simulink model "DC_motor_with_nested_PID"  (R2013b)
settings: Solver=ode45  StartTime=0.0  StopTime=20  MaxStep=0.1  RelTol=1e-3
values from neighbouring files (symbols this model uses):
  J = 1.66e-5    (= 1.66e-05)    [RunMotorSim.m]    (also in RunMotorSim_OpenLoop.m)
  KD = 1.33e-8    (= 1.33e-08)    [RunMotorSim.m]    (also in RunMotorSim_OpenLoop.m)
  KT = 7.5e-3    (= 0.0075)    [RunMotorSim.m]    (also in RunMotorSim_OpenLoop.m)
  pow = 1.88    [RunMotorSim.m]    (also in RunMotorSim_OpenLoop.m = 2)
libraries: simulink x1
settings Model: Creator=aberger  LastModifiedBy=aberger
settings DataIOCC: MaxDataPoints=100000

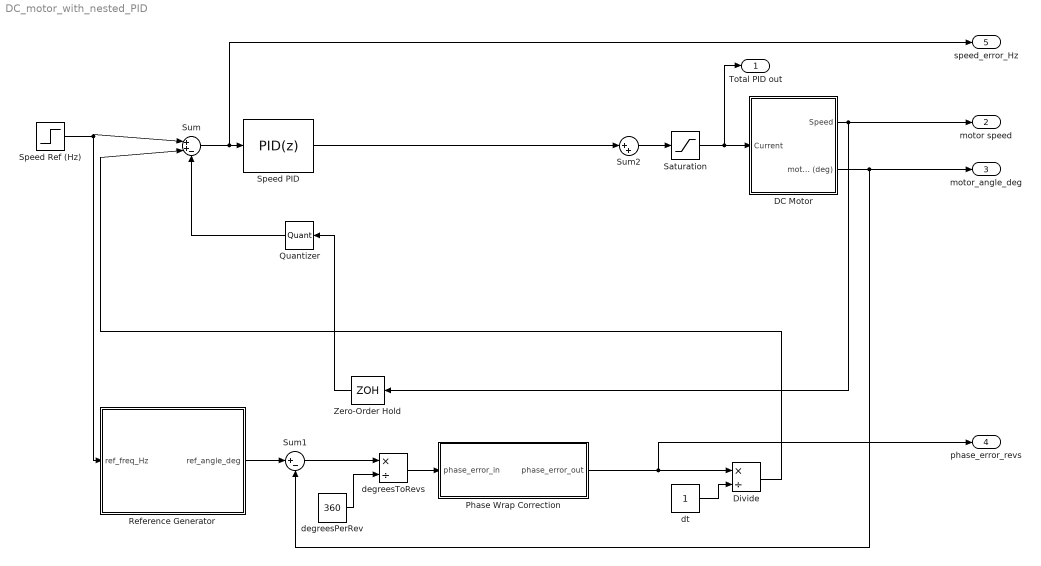
== system DC_motor_with_nested_PID ==
  DC Motor : Subsystem
  Divide : Product  Inputs=*/
  Phase Wrap Correction : Subsystem
  Quantizer : Quantizer  QuantizationInterval=.025
  Reference Generator : Subsystem
  Saturation : Saturate  UpperLimit=1  LowerLimit=0
  Speed PID : simulink/Continuous/PID Controller  Controller=PID  TimeDomain=Discrete-time  SampleTime=.001  IntegratorMethod=Forward Euler  FilterMethod=Forward Euler  Form=Parallel  P=0.4  I=.04  D=0  N=100  InitialConditionSource=internal  InitialConditionForIntegrator=0  InitialConditionForFilter=0  ExternalReset=none  LimitOutput=on  UpperSaturationLimit=1  LowerSaturationLimit=0  LinearizeAsGain=on  AntiWindupMode=none  Kb=1  TrackingMode=off  Kt=1  PParamMin=[]  PParamMax=[]  IParamMin=[]  IParamMax=[]  DParamMin=[]  DParamMax=[]  NParamMin=[]  NParamMax=[]  KbParamMin=[]  KbParamMax=[]  KtParamMin=[]  KtParamMax=[]  POutMin=[]  POutMax=[]  IOutMin=[]  IOutMax=[]  DOutMin=[]  DOutMax=[]  NOutMin=[]  NOutMax=[]  KbOutMin=[]  KbOutMax=[]  KtOutMin=[]  KtOutMax=[]  IntegratorOutMin=[]  IntegratorOutMax=[]  FilterOutMin=[]  FilterOutMax=[]  SumOutMin=[]  SumOutMax=[]  SumI1OutMin=[]  SumI1OutMax=[]  SumI2OutMin=[]  SumI2OutMax=[]  SumI3OutMin=[]  SumI3OutMax=[]  SumDOutMin=[]  SumDOutMax=[]  SaturationOutMin=[]  SaturationOutMax=[]  IntegratorContinuousStateAttributes=''  IntegratorStateMustResolveToSignalObject=off  IntegratorRTWStateStorageClass=Auto  FilterContinuousStateAttributes=''  FilterStateMustResolveToSignalObject=off  FilterRTWStateStorageClass=Auto
  Speed Ref (Hz) : Step  Time=4  After=50  SampleTime=0
  Sum : Sum  Inputs=|++-
  Sum1 : Sum  Inputs=|+-
  Sum2 : Sum  Inputs=|++
  Zero-Order Hold : ZeroOrderHold  SampleTime=.001
  degreesPerRev : Constant  Value=360
  degreesToRevs : Product  Inputs=*/
  dt : Constant
  Total PID out : Outport
  motor speed : Outport  Port=2
  motor_angle_deg : Outport  Port=3
  phase_error_revs : Outport  Port=4
  speed_error_Hz : Outport  Port=5
  wires:
  Sum/1 -> speed_error_Hz/1, Speed PID/1
  Speed Ref (Hz)/1 -> Reference Generator/1(ref_freq_Hz), Sum/1
  Speed PID/1 -> Sum2/1
  DC Motor/1(Speed) -> motor speed/1, Zero-Order Hold/1
  Zero-Order Hold/1 -> Quantizer/1
  Reference Generator/1(ref_angle_deg) -> Sum1/1
  Sum2/1 -> Saturation/1
  Saturation/1 -> Total PID out/1, DC Motor/1(Current)
  Sum1/1 -> degreesToRevs/1
  degreesPerRev/1 -> degreesToRevs/2
  DC Motor/2(motor angle (deg)) -> Sum1/2, motor_angle_deg/1
  degreesToRevs/1 -> Phase Wrap Correction/1(phase_error_in)
  Phase Wrap Correction/1(phase_error_out) -> Divide/1, phase_error_revs/1
  Quantizer/1 -> Sum/3
  dt/1 -> Divide/2
  Divide/1 -> Sum/2

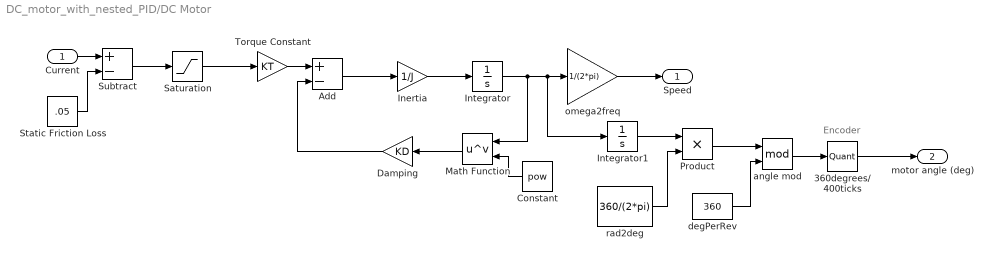
== system DC_motor_with_nested_PID/DC Motor ==
  note: Encoder
  Current : Inport
  "360degrees/ 400ticks " : Quantizer  QuantizationInterval=0.9
  Add : Sum  Inputs=+-
  Constant : Constant  Value=pow
  Damping : Gain  Gain=KD
  Inertia : Gain  Gain=1/J
  Integrator : Integrator
  Integrator1 : Integrator
  Math Function : Math  Operator=pow  SaturateOnIntegerOverflow=on
  Product : Product
  Saturation : Saturate  UpperLimit=1  LowerLimit=0
  Static Friction Loss : Constant  Value=.05
  Subtract : Sum  Inputs=+-
  Torque Constant : Gain  Gain=KT
  angle mod : Math  Operator=mod  SaturateOnIntegerOverflow=on
  degPerRev : Constant  Value=360
  omega2freq : Gain  Gain=1/(2*pi)
  rad2deg : Constant  Value=360/(2*pi)
  Speed : Outport
  motor angle (deg) : Outport  Port=2
  wires:
  Add/1 -> Inertia/1
  Integrator/1 -> Math Function/1, Integrator1/1, omega2freq/1
  Torque Constant/1 -> Add/1
  Damping/1 -> Add/2
  Inertia/1 -> Integrator/1
  Current/1 -> Subtract/1
  Constant/1 -> Math Function/2
  Math Function/1 -> Damping/1
  omega2freq/1 -> Speed/1
  Static Friction Loss/1 -> Subtract/2
  Integrator1/1 -> Product/1
  angle mod/1 -> "360degrees/ 400ticks "/1
  Product/1 -> angle mod/1
  rad2deg/1 -> Product/2
  degPerRev/1 -> angle mod/2
  Subtract/1 -> Saturation/1
  Saturation/1 -> Torque Constant/1
  "360degrees/ 400ticks "/1 -> motor angle (deg)/1

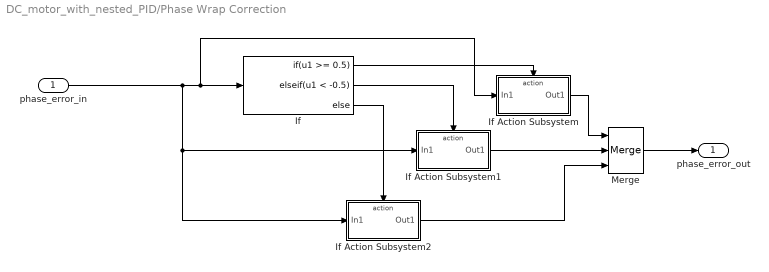
== system DC_motor_with_nested_PID/Phase Wrap Correction ==
  phase_error_in : Inport
  If : If  IfExpression=u1 >= 0.5  ElseIfExpressions=u1 < -0.5
  If Action Subsystem : Subsystem  TreatAsAtomicUnit=on
  If Action Subsystem1 : Subsystem  TreatAsAtomicUnit=on
  If Action Subsystem2 : Subsystem  TreatAsAtomicUnit=on
  Merge : Merge  Inputs=3
  phase_error_out : Outport
  wires:
  If/1 -> If Action Subsystem/Action
  If Action Subsystem/1(Out1) -> Merge/1
  If Action Subsystem2/1(Out1) -> Merge/3
  phase_error_in/1 -> If/1, If Action Subsystem/1(In1), If Action Subsystem1/1(In1), If Action Subsystem2/1(In1)
  If/2 -> If Action Subsystem1/Action
  If/3 -> If Action Subsystem2/Action
  Merge/1 -> phase_error_out/1
  If Action Subsystem1/1(Out1) -> Merge/2

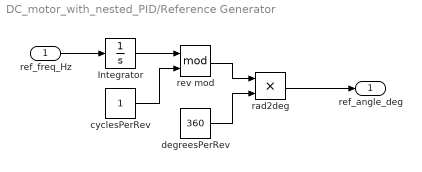
== system DC_motor_with_nested_PID/Reference Generator ==
  ref_freq_Hz : Inport
  Integrator : Integrator
  cyclesPerRev : Constant
  degreesPerRev : Constant  Value=360
  rad2deg : Product
  rev mod : Math  Operator=mod  SaturateOnIntegerOverflow=on
  ref_angle_deg : Outport
  wires:
  cyclesPerRev/1 -> rev mod/2
  degreesPerRev/1 -> rad2deg/2
  Integrator/1 -> rev mod/1
  rev mod/1 -> rad2deg/1
  rad2deg/1 -> ref_angle_deg/1
  ref_freq_Hz/1 -> Integrator/1

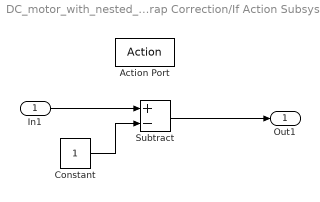
== system DC_motor_with_nested_PID/Phase Wrap Correction/If Action Subsystem ==
  In1 : Inport
  Action Port : ActionPort  ActionType=then
  Constant : Constant
  Subtract : Sum  Inputs=+-
  Out1 : Outport
  wires:
  In1/1 -> Subtract/1
  Constant/1 -> Subtract/2
  Subtract/1 -> Out1/1

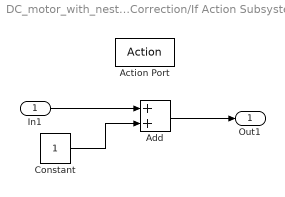
== system DC_motor_with_nested_PID/Phase Wrap Correction/If Action Subsystem1 ==
  In1 : Inport
  Action Port : ActionPort  ActionType=elseif
  Add : Sum
  Constant : Constant
  Out1 : Outport
  wires:
  In1/1 -> Add/1
  Constant/1 -> Add/2
  Add/1 -> Out1/1

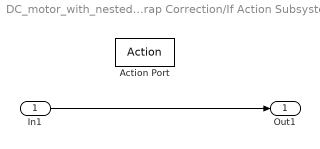
== system DC_motor_with_nested_PID/Phase Wrap Correction/If Action Subsystem2 ==
  In1 : Inport
  Action Port : ActionPort  ActionType=else
  Out1 : Outport
  wires:
  In1/1 -> Out1/1
